simulink model "m_0012_2_20"  (R2017a)
settings: Solver=ode3  StartTime=0  StopTime=InputData.TestData.Time_sec_(end)  FixedStep=0.01  RelTol=1e-3
values from neighbouring files (symbols this model uses):
  InputData = readtable(SimSetup.(fields{i}))    [DataProc_eff.m]
undefined symbols (not defined in the file or in its folder): Chassis, DiscIntNeverNeededParam, Ion, Lithium, Ptrain
libraries: powerlib x3, simulink x1, electricdrivelib x1
settings Model: Creator=TheCmak  LastModifiedBy=TheCmak

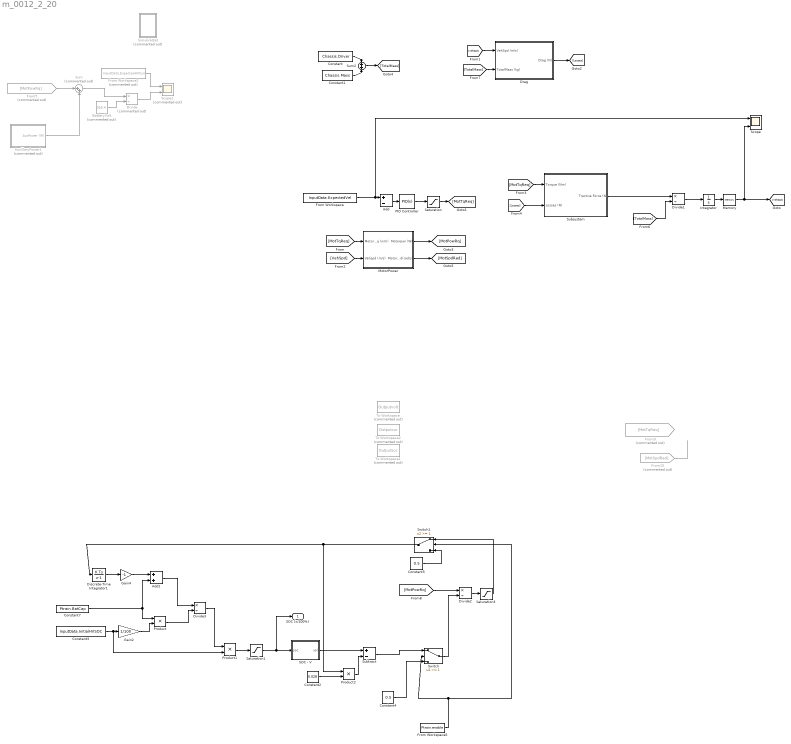
== system m_0012_2_20 ==
  Add : Sum  Inputs=+-
  Add1 : Sum
  AuxillaryPower1 : Subsystem  Commented=on
  BatteryVolt : Constant  Commented=on  Value=355.4
  Constant : Constant  Value=Chassis.Driver
  Constant1 : Constant  Value=Chassis.Mass
  Constant2 : Constant  Value=0.028
  Constant3 : Constant  Value=InputData.InitialHVSOC
  Constant4 : Constant  Value=0.5
  Constant5 : Constant  Value=0.5
  Constant7 : Constant  Value=Ptrain.BatCap
  Discrete-Time Integrator1 : DiscreteIntegrator  InitialCondition=Ptrain.BatCap-(Ptrain.BatCap*(InputData.InitialHVSOC/100))  InitialConditionSetting=State (most efficient)  SampleTime=-1  ICPrevOutput=DiscIntNeverNeededParam  ICPrevScaledInput=DiscIntNeverNeededParam
  Divide : Product  Commented=on  Inputs=*/
  Divide1 : Product  Inputs=*/
  Divide2 : Product  Inputs=*/
  Divide3 : Product  Inputs=*/
  Drag : Subsystem
  From Workspace : FromWorkspace  VariableName=InputData.ExpectedVel
  From Workspace2 : FromWorkspace  Commented=on  VariableName=InputData.ExpectedHVCurr  SampleTime=0
  From Workspace5 : FromWorkspace  VariableName=Ptrain.enable  SampleTime=0
  From10 : From  Commented=on  GotoTag=MotSpdRad
  From5 : From  Commented=on  GotoTag=MotPowRq
  From9 : From  Commented=on  GotoTag=MotTqReq
  Gain2 : Gain  Gain=1/100
  Gain4 : Gain  Gain=-1
  Integrator : Integrator
  Memory : Memory
  MotorPower : Subsystem
  PID Controller : simulink/Continuous/PID Controller  Controller=PID  TimeDomain=Continuous-time  SampleTime=-1  IntegratorMethod=Forward Euler  FilterMethod=Forward Euler  Form=Parallel  UseFilter=on  ControllerParametersSource=internal  P=350  I=0.0001  D=0  N=100  InitialConditionSource=internal  InitialConditionForIntegrator=0  InitialConditionForFilter=0  ExternalReset=none  LimitOutput=off  UpperSaturationLimit=inf  LowerSaturationLimit=-inf  LinearizeAsGain=on  AntiWindupMode=none  Kb=1  TrackingMode=off  Kt=1  PParamMin=[]  PParamMax=[]  IParamMin=[]  IParamMax=[]  DParamMin=[]  DParamMax=[]  NParamMin=[]  NParamMax=[]  KbParamMin=[]  KbParamMax=[]  KtParamMin=[]  KtParamMax=[]  POutMin=[]  POutMax=[]  IOutMin=[]  IOutMax=[]  DOutMin=[]  DOutMax=[]  NOutMin=[]  NOutMax=[]  KbOutMin=[]  KbOutMax=[]  KtOutMin=[]  KtOutMax=[]  IntegratorOutMin=[]  IntegratorOutMax=[]  FilterOutMin=[]  FilterOutMax=[]  SumOutMin=[]  SumOutMax=[]  SumI1OutMin=[]  SumI1OutMax=[]  SumI2OutMin=[]  SumI2OutMax=[]  SumI3OutMin=[]  SumI3OutMax=[]  SumDOutMin=[]  SumDOutMax=[]  SaturationOutMin=[]  SaturationOutMax=[]  IntegratorContinuousStateAttributes=''  IntegratorStateMustResolveToSignalObject=off  IntegratorRTWStateStorageClass=Auto  FilterContinuousStateAttributes=''  FilterStateMustResolveToSignalObject=off  FilterRTWStateStorageClass=Auto  DifferentiatorICPrevScaledInput=0  DifferentiatorOutMin=[]  DifferentiatorOutMax=[]  InitialConditionSetting=State (most efficient)
  Product : Product
  Product1 : Product
  Product2 : Product
  SOC - V : MATLAB Function  TreatAsAtomicUnit=on
  Saturation : Saturate  UpperLimit=444  LowerLimit=-200
  Saturation1 : Saturate  UpperLimit=100  LowerLimit=0
  Saturation3 : Saturate  UpperLimit=1000  LowerLimit=-1000
  Scope : Scope  NumInputPorts=2
  Scope1 : Scope  Commented=on  NumInputPorts=2
  "SimulinkBat " : Subsystem  Commented=on
  Subsystem : Subsystem
  Subtract : Sum  Inputs=+-
  Sum : Sum  Commented=on  Inputs=|++
  Sum2 : Sum  Inputs=2
  Switch : Switch  Threshold=1
  Switch1 : Switch  Threshold=1
  To Workspace : ToWorkspace  Commented=on  VariableName=Outputvolt  SaveFormat=Timeseries  SampleTime=InputData.SampleRate
  To Workspace1 : ToWorkspace  Commented=on  VariableName=Outputsoc  SaveFormat=Timeseries  SampleTime=InputData.SampleRate
  To Workspace2 : ToWorkspace  Commented=on  VariableName=Outputcur  SaveFormat=Timeseries  SampleTime=InputData.SampleRate
  SOC (x/100%) : Outport
  wires:
  From Workspace/1 -> Scope/1, Add/1
  Add/1 -> PID Controller/1
  Integrator/1 -> Memory/1
  [TotalMass] -> Divide1/2
  PID Controller/1 -> Saturation/1
  Memory/1 -> Scope/2, [VehSpd]
  Saturation/1 -> [MotTqReq]
  [MotTqReq] -> MotorPower/1(MotorTq (n/m))
  [VehSpd] -> MotorPower/2("Vehspd (m/s) ")
  [VehSpd] -> Drag/1(VehSpd (m/s))
  MotorPower/1(Motorpwr (W)) -> [MotPowRq]
  Divide1/1 -> Integrator/1
  Drag/1(Drag (N)) -> [Losses]
  [MotTqReq] -> Subsystem/1(Torque (Nm))
  [Losses] -> Subsystem/2(Losses (N))
  Subsystem/1(Tractive Force (N)) -> Divide1/1
  From5/1 -> Sum/1
  BatteryVolt/1 -> Divide/2
  AuxillaryPower1/1(AuxPower (W)) -> Sum/2
  Sum/1 -> Divide/1
  From Workspace2/1 -> Scope1/1
  Divide/1 -> Scope1/2
  Constant/1 -> Sum2/1
  Constant1/1 -> Sum2/2
  Sum2/1 -> [TotalMass]
  [TotalMass] -> Drag/2("TotalMass (kg) ")
  Divide2/1 -> Saturation3/1
  Discrete-Time Integrator1/1 -> Gain4/1
  Gain2/1 -> Product/2
  Switch1/1 -> Product2/1, Discrete-Time Integrator1/1
  Product1/1 -> Saturation1/1
  Add1/1 -> Divide3/1
  Saturation3/1 -> Switch1/1
  Constant5/1 -> Switch1/3
  From Workspace5/1 -> Switch/2, Switch1/2
  Constant4/1 -> Switch/3
  Saturation1/1 -> SOC (x/100%)/1, SOC - V/1(soc)
  Constant3/1 -> Product1/2, Gain2/1
  [MotPowRq] -> Divide2/1
  SOC - V/1(vol) -> Subtract/1
  Subtract/1 -> Switch/1
  Switch/1 -> Divide2/2
  Constant2/1 -> Product2/2
  Constant7/1 -> Product/1, Add1/2
  Gain4/1 -> Add1/1
  Product2/1 -> Subtract/2
  Divide3/1 -> Product1/1
  Product/1 -> Divide3/2
  MotorPower/2("MotorSpd(rad/s) ") -> [MotSpdRad]
  From10/1 -> ?

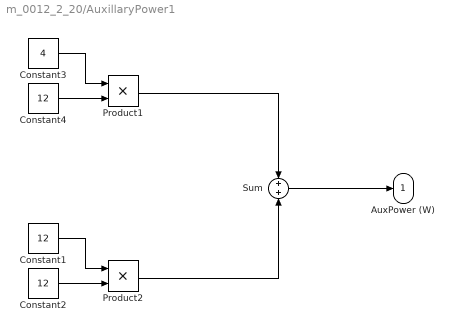
== system m_0012_2_20/AuxillaryPower1 ==
  Constant1 : Constant  Value=12
  Constant2 : Constant  Value=12
  Constant3 : Constant  Value=4
  Constant4 : Constant  Value=12
  Product1 : Product
  Product2 : Product
  Sum : Sum  Inputs=2
  AuxPower (W) : Outport
  wires:
  Product2/1 -> Sum/2
  Constant1/1 -> Product2/1
  Constant2/1 -> Product2/2
  Sum/1 -> AuxPower (W)/1
  Constant4/1 -> Product1/2
  Constant3/1 -> Product1/1
  Product1/1 -> Sum/1

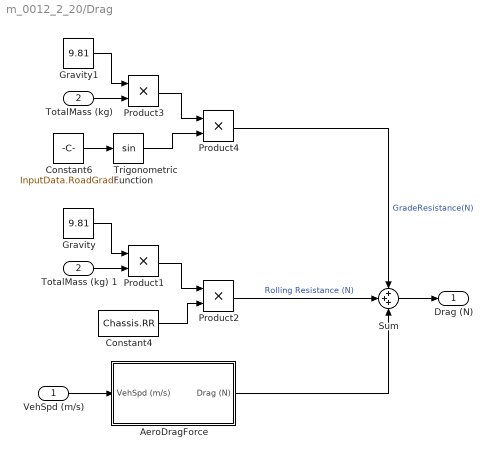
== system m_0012_2_20/Drag ==
  VehSpd (m/s) : Inport
  "TotalMass (kg) " : Inport  Port=2
  AeroDragForce : Subsystem
  Constant4 : Constant  Value=Chassis.RR
  Constant6 : Constant  Value=InputData.RoadGrade
  Gravity : Constant  Value=9.81
  Gravity1 : Constant  Value=9.81
  Product{1..4} (4 alike) : Product
  Sum : Sum  Inputs=3
  TotalMass (kg) 1 : InportShadow  Port=2
  Trigonometric Function : Trigonometry
  Drag (N) : Outport
  wires:
  Gravity/1 -> Product1/1
  Product3/1 -> Product4/1
  Gravity1/1 -> Product3/1
  "TotalMass (kg) "/1 -> Product3/2
  Trigonometric Function/1 -> Product4/2
  Product1/1 -> Product2/1
  Constant4/1 -> Product2/2
  Constant6/1 -> Trigonometric Function/1
  Product4/1 -> Sum/1  "GradeResistance(N)"
  AeroDragForce/1(Drag (N)) -> Sum/3
  Product2/1 -> Sum/2  "Rolling Resistance (N)"
  TotalMass (kg) 1/1 -> Product1/2
  VehSpd (m/s)/1 -> AeroDragForce/1(VehSpd (m/s))
  Sum/1 -> Drag (N)/1

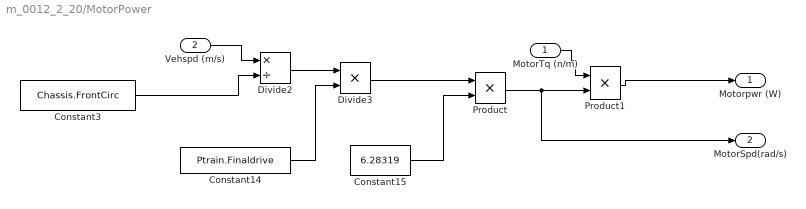
== system m_0012_2_20/MotorPower ==
  MotorTq (n/m) : Inport
  "Vehspd (m/s) " : Inport  Port=2
  Constant14 : Constant  Value=Ptrain.Finaldrive
  Constant15 : Constant  Value=6.28319
  Constant3 : Constant  Value=Chassis.FrontCirc
  Divide2 : Product  Inputs=*/
  Divide3 : Product  Inputs=**
  Product : Product
  Product1 : Product
  Motorpwr (W) : Outport
  "MotorSpd(rad/s) " : Outport  Port=2
  wires:
  MotorTq (n/m)/1 -> Product1/1
  "Vehspd (m/s) "/1 -> Divide2/1
  Constant3/1 -> Divide2/2
  Product/1 -> "MotorSpd(rad/s) "/1, Product1/2
  Divide2/1 -> Divide3/1
  Product1/1 -> Motorpwr (W)/1
  Constant14/1 -> Divide3/2
  Divide3/1 -> Product/1
  Constant15/1 -> Product/2

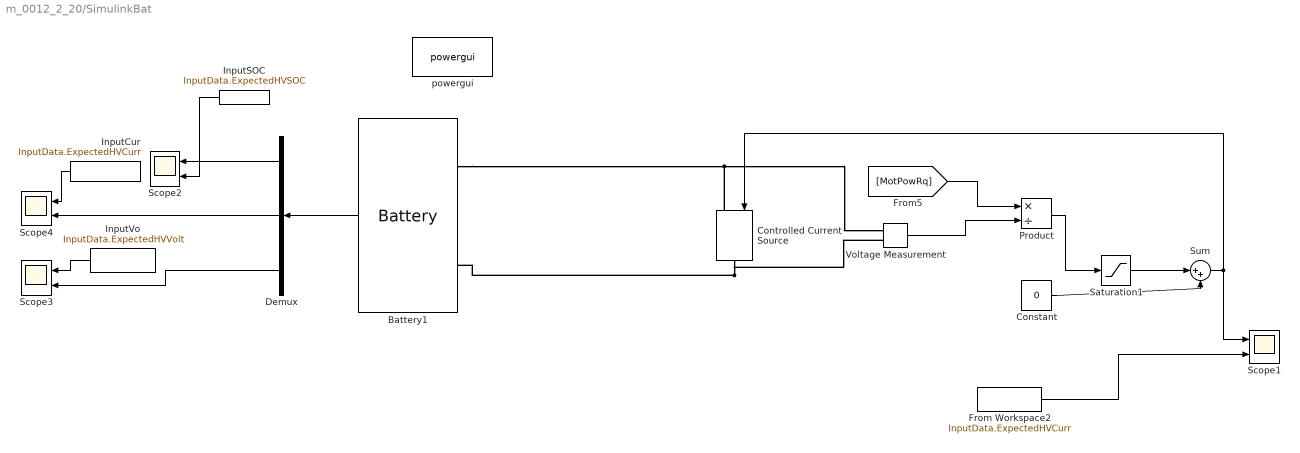
== system m_0012_2_20/SimulinkBat  ==
  Battery1 : electricdrivelib/Extra Sources/Battery  BatType=Lithium-Ion  ShowTempParam=off  ThermalPreset=no  ShowAgeParam=off  NomV=355.2  NomQ=52  SOC=InputData.InitialHVSOC  Batt_Tr=0.01  PresetModel=off  MaxQ=52  MinV=288  FullV=398.4  Dis_rate=300  R=0.1  Normal_OP=47.0261  expZone="[383.7531      2.554783]"  current=[6.5 13 32.5]  Units=Time  Tci=20  NomT=20  T2=-30  MaxQ2=4.8  FullV2=7.1  Normal_OP2=5.655  expZone2="[6.58           1]"  Rca=0.6  ti=2000  Dp=0  Neq0=0  Tsim=1e6  Ta1=25  Qeol=5.4*0.9  Reol=0.013333*1.2  Char_age=[2.3478, 3]  Dis_age=[2.3478, 10]  N1=1500  N2=10500  N3=1000  N4=1400  Ta2=45  N5=950
  Constant : Constant  Value=0
  Controlled Current Source : powerlib/Electrical Sources/Controlled Current Source  Initialize=on  Source_Type=DC  Amplitude=0  Phase=0  Frequency=0  Measurements=None
  Demux : Demux  Outputs=3
  From Workspace2 : FromWorkspace  VariableName=InputData.ExpectedHVCurr  SampleTime=0
  "InputCur " : FromWorkspace  VariableName=InputData.ExpectedHVCurr  SampleTime=0
  InputSOC : FromWorkspace  VariableName=InputData.ExpectedHVSOC  SampleTime=0
  InputVo : FromWorkspace  VariableName=InputData.ExpectedHVVolt  SampleTime=0
  Product : Product  Inputs=*/
  Saturation1 : Saturate  UpperLimit=444  LowerLimit=-200
  Scope{1..4} (4 alike) : Scope  NumInputPorts=2
  Sum : Sum  Inputs=|++
  Voltage Measurement : powerlib/Measurements/Voltage Measurement  PhasorSimulation=off  OutputType=Complex  PSBequivalent=0
  powergui : powerlib/powergui  Priority=1  SimulationMode=Discrete  SampleTime=0.01  frequency=60  Iterations=50  frequencyindice=0  Pbase=100e6  ErrMax=1e-4  UnitsV=kV  UnitsW=MW  buscounter=0  FunctionMessages=off  echomessages=off  EnableUseOfTLC=off  CurrentSourceSwitches=off  DisableSnubberDevices=off  DisableRonSwitches=off  DisableVfSwitches=off  DisplayEquations=off  SolverType=Tustin/Backward Euler (TBE)  Interpol=off  ExternalGateDelay=off  methode=off  Ts=100  x0status=blocks  SPID=on  SwTol=0  HookPort=off  RestoreLinks=warning  ResistiveCurrentMeasurement=off  Frange=[0:2:500]  Ylog=off  Xlog=on  ShowGrid=off  save=off  variable=ZData  structure=0  ZoomFFT=off  StartTime=0.0  cycles=1  DisplayStyle=1  fundamental=60  FreqAxis=off  MaxFrequency=1000  frequencyindicesteady=1  RmsSteady=1  display=off
  wires:
  Battery1/1 -> Demux/1
  Product/1 -> Saturation1/1
  Demux/2 -> Scope4/2
  Demux/3 -> Scope3/2
  InputVo/1 -> Scope3/1
  From Workspace2/1 -> Scope1/2
  Demux/1 -> Scope2/1
  Constant/1 -> Sum/2
  Voltage Measurement/1 -> Product/2
  Sum/1 -> Controlled Current Source/1, Scope1/1
  Saturation1/1 -> Sum/1
  "InputCur "/1 -> Scope4/1
  [MotPowRq] -> Product/1
  InputSOC/1 -> Scope2/2
  connections:
  Battery1/LConn2 -- Voltage Measurement/LConn2 -- Controlled Current Source/RConn1
  Battery1/LConn1 -- Voltage Measurement/LConn1 -- Controlled Current Source/LConn1

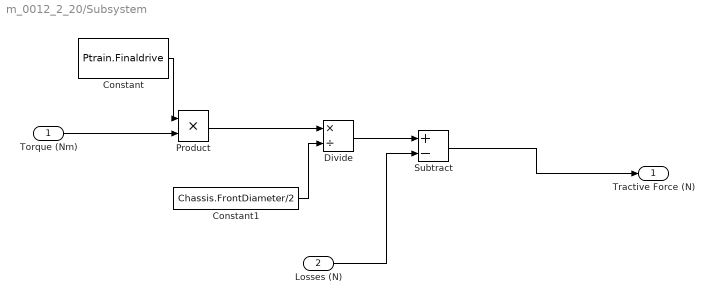
== system m_0012_2_20/Subsystem ==
  Torque (Nm) : Inport
  Losses (N) : Inport  Port=2
  Constant : Constant  Value=Ptrain.Finaldrive
  Constant1 : Constant  Value=Chassis.FrontDiameter/2
  Divide : Product  Inputs=*/
  Product : Product
  Subtract : Sum  Inputs=+-
  Tractive Force (N) : Outport
  wires:
  Torque (Nm)/1 -> Product/2
  Constant1/1 -> Divide/2
  Product/1 -> Divide/1
  Constant/1 -> Product/1
  Divide/1 -> Subtract/1
  Subtract/1 -> Tractive Force (N)/1
  Losses (N)/1 -> Subtract/2

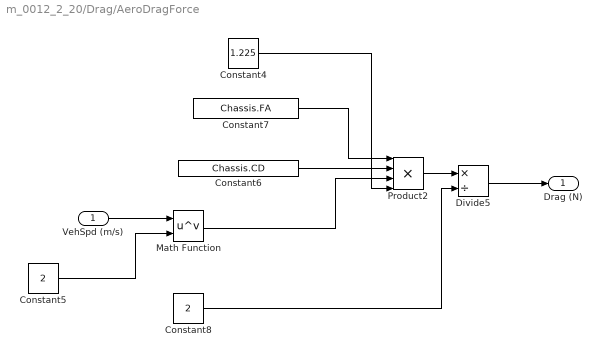
== system m_0012_2_20/Drag/AeroDragForce ==
  VehSpd (m/s) : Inport
  Constant4 : Constant  Value=1.225
  Constant5 : Constant  Value=2
  Constant6 : Constant  Value=Chassis.CD
  Constant7 : Constant  Value=Chassis.FA
  Constant8 : Constant  Value=2
  Divide5 : Product  Inputs=*/
  Math Function : Math  Operator=pow  SaturateOnIntegerOverflow=on
  Product2 : Product  Inputs=4
  Drag (N) : Outport
  wires:
  Product2/1 -> Divide5/1
  Constant7/1 -> Product2/1
  Constant5/1 -> Math Function/2
  Constant6/1 -> Product2/2
  Math Function/1 -> Product2/3
  Constant4/1 -> Product2/4
  Constant8/1 -> Divide5/2
  Divide5/1 -> Drag (N)/1
  VehSpd (m/s)/1 -> Math Function/1

== matlab function m_0012_2_20/SOC - V ==
  data: soc input; vol output
function vol = f(soc)
    a = 330.5;
    b = 0.001814;
    c = -72.16;
    d = -0.4065;
    expvol = a*exp(b*soc) + c*exp(d*soc);
vol = expvol;
